simulink model "dcl_ut"  (Simulink 8.1)
settings: Solver=FixedStepDiscrete  StartTime=0.0  StopTime=Inf  FixedStep=0.001  RelTol=1e-3
PostLoadFcn:
  | , if any(exist('dsrtsu_mdlpostloadfcn', 'file') == [2, 3, 6]), try dsrtsu_mdlpostloadfcn('Execute', bdroot); catch fprintf('Error in PostLoadFcn (dsrtsu_mdlpostloadfcn) for model "%s":\n %s\n', bdroot, lasterr); end, end,
libraries: siltestlib x18, dcl x1
settings Model: DSRTSU_INTERNAL_RTI_VER=450  DSRTSU_INTERNAL_RTI_TYPE=rti1401  RTICANMMDATA=struct('GeneralSetupData',struct('modelroot','D:\ELN150201_TAIWAN\trunk\AdasDragon\software\sw_development\arch\app\acc','generalsettings',struct('filesettings',struct('destfolder',struct('Name','RTICANMM_FILES','Check',1),'buildfolder',struct('Name','.','Check',1),'AbsDestfolder',struct('Name','D:\ELN150201_TAIWAN\trunk\AdasDragon\software\sw_development\arch\app\acc\RTICANMM_FILES'),'AbsBuildfolder',struct('Name','D:\ELN150201_TAIWAN\trunk\AdasDragon\software\sw_development\arch\app\acc'))),'options',struct('addpaths',1,'rmpaths',1,'addtrcexclusion',logical(1),'cannavigator',struct('checkmonitoring',0),'show_usrtrc',0,'use_usrtrc',0),'advanced',struct('options',[1 1 1 1 1 1 1 1 1 1 1 1 1 1 1 1 1 1 1 1 1 1 1 1 1 1 1 1 1 1 1 1 1 1 1 1 1 1 1 1 1 1 1 1 1 1 1 1 1 1 1 1 1 1 1 1 1 1 1 1 1 1 1 1 1 1 1 1 1 1 1 1 1 1 1 1 1 1 1 1 1 1 1 1 1 1 1 1 1 1 1 1 1 1 1 1 1 1 1 1]),'MPSetup',{{}},'modelname','dcl_ut','block','dcl_ut'))  DSRTSU_INTERNAL_RTIFPGA=40  Creator=AT015411  LastModifiedBy=AT015555  BufferReuse=off
settings DataIOCC: SignalLoggingSaveFormat=Dataset
settings OptimizationCC: BlockReduction=off  OptimizeBlockIOStorage=off  BufferReuse=off  ExpressionFolding=off  ExpressionDepthLimit=128  LocalBlockOutputs=off
settings DebuggingCC: FcnCallInpInsideContextMsg=EnableAllAsError
settings HardwareCC: ProdIntDivRoundTo=Zero  ProdEndianess=BigEndian  ProdHWDeviceType=Generic->Custom  TargetIntDivRoundTo=Zero  TargetEndianess=BigEndian  TargetHWDeviceType=Generic->Custom
settings RTWCC: SystemTargetFile=rti1005.tlc  MakeCommand=make_rti  TemplateMakefile=rti1005.tmf  Description=dSPACE DS1005 Hardware Platform  ProcessScript=rti1005_make_rtw_hook
settings STFCustomTargetCC: CodeReplacementLibrary=ANSI_C  ParMdlRefBuildCompliant=on  GeneratePreprocessorConditionals=Disable all  MatFileLogging=on  SystemTargetFile=rti1005.tlc
settings GRTTargetCC: CompOptLevelCompliant=off  ConcurrentExecutionCompliant=off  ExtModeMexFile=noextcomm
settings CustomProperty: DataType=RTWOptions_EnumType_C__Program Files (x86)_dSPACE RCPHIL 2014-B_MATLAB_RTI_RTI1401_TLC_rti1005_1InitialSimState  Value=RUN
settings EnumStrPairs: String=RUN

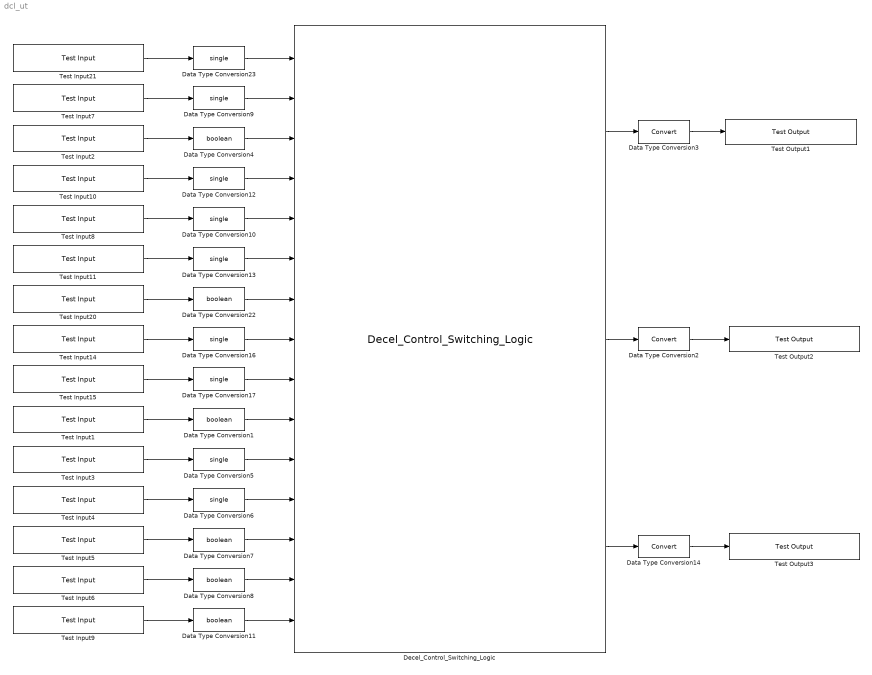
== system dcl_ut ==
  Data Type Conversion{1,4,7..8,11,22} (6 alike) : DataTypeConversion  OutDataTypeStr=boolean
  Data Type Conversion{5..6,9..10,12..13,16..17,23} (9 alike) : DataTypeConversion  OutDataTypeStr=single
  Data Type Conversion14 : DataTypeConversion
  Data Type Conversion2 : DataTypeConversion
  Data Type Conversion3 : DataTypeConversion
  Decel_Control_Switching_Logic : dcl/Decel_Control_Switching_Logic
  Test Input1 : siltestlib/Test Input  varname=VACC_ACCOverride_flg  sampletime=0.005
  Test Input10 : siltestlib/Test Input  varname=VIFO_ACCVehClearance_m  sampletime=0.005
  Test Input11 : siltestlib/Test Input  varname=VIFO_ACCTargetVehRelSpeedX_mps  sampletime=0.005
  Test Input14 : siltestlib/Test Input  varname=VJUD_ACCSetTimeGap_s  sampletime=0.005
  Test Input15 : siltestlib/Test Input  varname=VIFO_ACCTGap_s  sampletime=0.005
  Test Input2 : siltestlib/Test Input  varname=VIFO_ACCDistControlSel_flg  sampletime=0.005
  Test Input20 : siltestlib/Test Input  varname=VACC_ACCTargetVehAssigned_flg  sampletime=0.005
  Test Input21 : siltestlib/Test Input  varname=VACC_ACCRefSpd_mps  sampletime=0.005
  Test Input3 : siltestlib/Test Input  varname=VACC_ACCMCDecel_mps2  sampletime=0.005
  Test Input4 : siltestlib/Test Input  varname=VACC_ACCTargetVehSpd_mps  sampletime=0.005
  Test Input5 : siltestlib/Test Input  varname=VACC_ACCTransitory_flg  sampletime=0.005
  Test Input6 : siltestlib/Test Input  varname=VACC_ACCMCBraking_flg  sampletime=0.005
  Test Input7 : siltestlib/Test Input  varname=VACC_DesiredDistance_m  sampletime=0.005
  Test Input8 : siltestlib/Test Input  varname=VACC_VehSpd_mps  sampletime=0.005
  Test Input9 : siltestlib/Test Input  varname=VACC_ACCBrakeToStop_flg  sampletime=0.005
  Test Output1 : siltestlib/Test Output  varname=VACC_DecelControlReq_flg  sampletime=-1
  Test Output2 : siltestlib/Test Output  varname=VACC_TorqueReleaseReq_flg  sampletime=-1
  Test Output3 : siltestlib/Test Output  varname=VACC_ACCBrakeReleaseSituation_flg  sampletime=-1
  wires:
  Data Type Conversion2/1 -> Test Output2/1
  Decel_Control_Switching_Logic/2 -> Data Type Conversion2/1
  Data Type Conversion3/1 -> Test Output1/1
  Decel_Control_Switching_Logic/1 -> Data Type Conversion3/1
  Test Input7/1 -> Data Type Conversion9/1
  Data Type Conversion9/1 -> Decel_Control_Switching_Logic/2
  Test Input8/1 -> Data Type Conversion10/1
  Test Input10/1 -> Data Type Conversion12/1
  Test Input11/1 -> Data Type Conversion13/1
  Test Input14/1 -> Data Type Conversion16/1
  Test Input15/1 -> Data Type Conversion17/1
  Test Input20/1 -> Data Type Conversion22/1
  Test Input21/1 -> Data Type Conversion23/1
  Data Type Conversion23/1 -> Decel_Control_Switching_Logic/1
  Test Input1/1 -> Data Type Conversion1/1
  Test Input2/1 -> Data Type Conversion4/1
  Data Type Conversion4/1 -> Decel_Control_Switching_Logic/3
  Data Type Conversion10/1 -> Decel_Control_Switching_Logic/5
  Data Type Conversion13/1 -> Decel_Control_Switching_Logic/6
  Data Type Conversion22/1 -> Decel_Control_Switching_Logic/7
  Data Type Conversion17/1 -> Decel_Control_Switching_Logic/9
  Data Type Conversion1/1 -> Decel_Control_Switching_Logic/10
  Data Type Conversion12/1 -> Decel_Control_Switching_Logic/4
  Data Type Conversion16/1 -> Decel_Control_Switching_Logic/8
  Test Input3/1 -> Data Type Conversion5/1
  Data Type Conversion5/1 -> Decel_Control_Switching_Logic/11
  Test Input4/1 -> Data Type Conversion6/1
  Data Type Conversion6/1 -> Decel_Control_Switching_Logic/12
  Test Input5/1 -> Data Type Conversion7/1
  Test Input6/1 -> Data Type Conversion8/1
  Test Input9/1 -> Data Type Conversion11/1
  Data Type Conversion7/1 -> Decel_Control_Switching_Logic/13
  Data Type Conversion11/1 -> Decel_Control_Switching_Logic/15
  Data Type Conversion8/1 -> Decel_Control_Switching_Logic/14
  Data Type Conversion14/1 -> Test Output3/1
  Decel_Control_Switching_Logic/3 -> Data Type Conversion14/1
